simulink library "two_state_button"  (R2023b)
settings: Solver=VariableStepAuto  StartTime=0.0  StopTime=10.0  RelTol=1e-3
libraries: simulink_extras x1
settings Model: Creator=mueller.chris-it22  LastModifiedBy=mueller.chris-it22

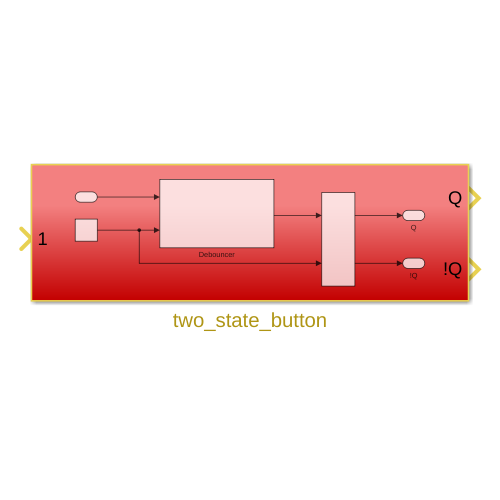
[thumbnail: Simulink's stored preview of the top-level diagram]
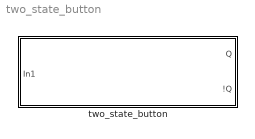
== system two_state_button ==
  two_state_button : Subsystem

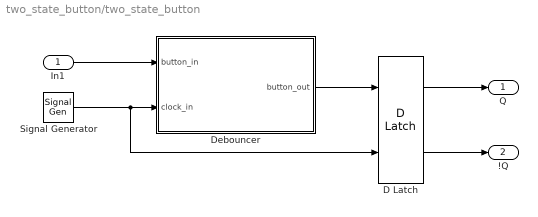
== system two_state_button/two_state_button ==
  In1 : Inport  OutDataTypeStr=boolean
  D Latch : simulink_extras/Flip Flops/D Latch
  Debouncer : MATLAB Function  TreatAsAtomicUnit=on
  Signal Generator : SignalGenerator  WaveForm=square  Frequency=1000
  Q : Outport  OutDataTypeStr=boolean
  !Q : Outport  Port=2
  wires:
  D Latch/2 -> !Q/1
  D Latch/1 -> Q/1
  Debouncer/1(button_out) -> D Latch/1
  In1/1 -> Debouncer/1(button_in)
  Signal Generator/1 -> Debouncer/2(clock_in), D Latch/2

== matlab function two_state_button/Debouncer ==
  data: button_in input; button_out output; clock_in input
function button_out = debounce(button_in, clock_in)
% DEBOUNCE: Entprellt einen Button-Eingang
% Inputs:
%   button_in - Boolescher Eingang (1 = gedrückt, 0 = nicht gedrückt)
%   clock_in  - Clock-Takt (1000 Hz, entspricht 1 ms pro Tick)
% Output:
%   button_out - Entprellter Button-Ausgang (1 = gedrückt, 0 = nicht gedrückt)

% Persistent Variable für den Timer und Zustand
persistent timer button_state

% Initialisierung bei erster Ausführung
if isempty(timer)
    timer = 0;          % Timer startet bei 0
    button_state = 0;   % Ausgangszustand ist "nicht gedrückt"
end

% Wenn der Button gedrückt ist, Timer erhöhen
if button_in
    timer = timer + 1;
    if timer >= DeboucneTime % 100 ms = 100 Ticks bei 100 Hz Clock
        button_state = 1; % Button ist stabil gedrückt
    end
else
    % Wenn Button losgelassen wird, Timer zurücksetzen
    timer = 0;
    button_state = 0; % Button ist nicht gedrückt
end

% Ausgabe des entprellten Signals
button_out = button_state;
end
